simulink model "SEGWAY_SIM_PID"  (R2018a)
settings: Solver=ode23t  StartTime=0.0  StopTime=5  FixedStep=ts  RelTol=1e-6  AbsTol=1e-9
values from neighbouring files (symbols this model uses):
  param = [M m Ith Imr h W R Ke Rm Trmax Dm n]    [CONTROL_SEGWAY.m]
  X0 = [0 0 th0*pi/180]'    [CONTROL_SEGWAY.m]
undefined symbols (not defined in the file or in its folder): K, matA, matB, matC, matD, Td, Ti
settings Model: ExtModeTrigMode=oneshot  ExtModeArmWhenConnect=off  Creator=zamora  LastModifiedBy=zamora
settings SolverCC: AutoScaleAbsTol=off  ZeroCrossControl=EnableAll  ZeroCrossAlgorithm=Adaptive
settings DataIOCC: SaveFormat=Array  SignalLoggingSaveFormat=ModelDataLogs  SaveOutput=off  SaveTime=off  StateSaveName=x  TimeSaveName=t  OutputSaveName=y
settings OptimizationCC: BlockReduction=off  BooleanDataType=off  DefaultParameterBehavior=Inlined  BufferReuse=off  ExpressionDepthLimit=2147483647  LifeSpan=inf
settings DebuggingCC: SaveWithParameterizedLinksMsg=none  UnderspecifiedInitializationDetection=Classic  MergeDetectMultiDrivingBlocksExec=none  SignalResolutionControl=TryResolveAllWithWarning  MaxConsecutiveZCsMsg=none  IgnoredZcDiagnostic=none  MultiTaskDSMMsg=warning  MultiTaskCondExecSysMsg=none  FcnCallInpInsideContextMsg=warning  StateNameClashWarn=warning  SFUnexpectedBacktrackingDiag=warning  SFNoUnconditionalDefaultTransitionDiag=warning  SFExecutionAtInitializationDiag=none
settings HardwareCC: ProdBitPerPointer=32  ProdBitPerSizeT=32  ProdBitPerPtrDiffT=32  ProdLargestAtomicFloat=None  ProdIntDivRoundTo=Undefined  ProdEndianess=Unspecified  ProdWordSize=32  ProdHWDeviceType=32-bit Generic  TargetBitPerPointer=64  TargetBitPerSizeT=64  TargetBitPerPtrDiffT=64  TargetLongLongMode=on  TargetIntDivRoundTo=Zero  TargetEndianess=LittleEndian  TargetWordSize=64  TargetHWDeviceType=MATLAB Host  ProdEqTarget=off
settings ModelReferenceCC: PropagateSignalLabelsOutOfModel=off
settings RTWCC: TemplateMakefile=grt_unix.tmf
settings CodeAppCC: StateflowObjectComments=on
settings GRTTargetCC: TargetLangStandard=C89/C90 (ANSI)  GeneratePreprocessorConditionals=Disable all  CombineOutputUpdateFcns=off  GRTInterface=on
settings ConfigComp: CovMetricSettings=dw  CovHtmlReporting=on  CovSaveCumulativeToWorkspaceVar=on  CovSaveSingleToWorkspaceVar=on  CovExternalEMLEnable=off  CovSFcnEnable=off

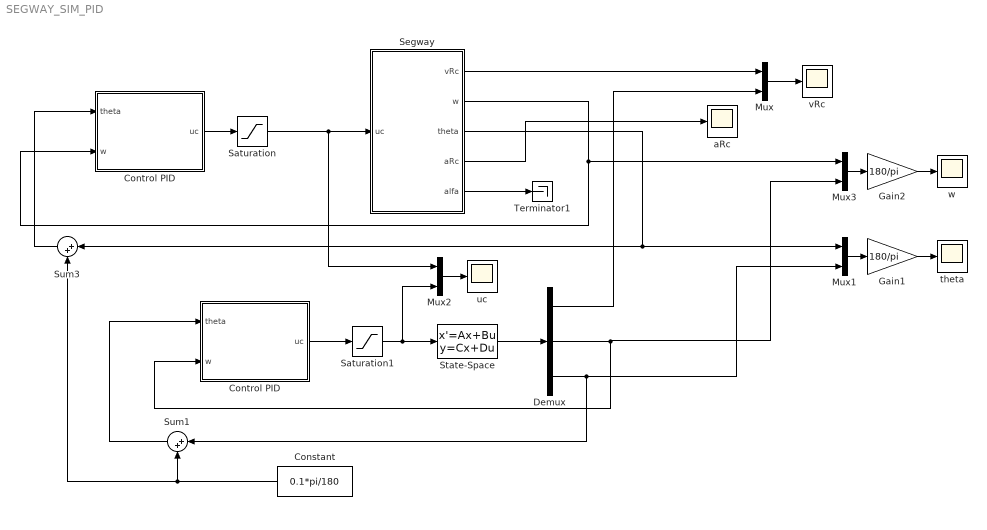
== system SEGWAY_SIM_PID ==
  Constant : Constant  Value=0.1*pi/180  SampleTime=0
  Control PID : Subsystem
  "Control PID " : Subsystem
  Demux : Demux  Outputs=3
  Gain1 : Gain  Gain=180/pi
  Gain2 : Gain  Gain=180/pi
  Mux{,1..3} (4 alike) : Mux  Inputs=2
  Saturation : Saturate  UpperLimit=8.5  LowerLimit=-8.5
  Saturation1 : Saturate  UpperLimit=8.5  LowerLimit=-8.5
  Segway : Subsystem
  State-Space : StateSpace  A=matA  B=matB  C=matC  D=matD  InitialCondition=X0
  Sum1 : Sum  Inputs=|++
  Sum3 : Sum  Inputs=|++
  Terminator1 : Terminator
  aRc : Scope
  theta : Scope
  uc : Scope
  vRc : Scope
  w : Scope
  wires:
  Gain1/1 -> theta/1
  Sum3/1 -> Control PID/1(theta)
  Control PID/1(uc) -> Saturation/1
  Segway/2(w) -> Control PID/2(w), Mux3/1
  Segway/5(alfa) -> Terminator1/1
  "Control PID "/1(uc) -> Saturation1/1
  Sum1/1 -> "Control PID "/1(theta)
  State-Space/1 -> Demux/1
  Demux/3 -> Mux1/2, Sum1/1
  Demux/2 -> Mux3/2, "Control PID "/2(w)
  Mux/1 -> vRc/1
  Mux1/1 -> Gain1/1
  Segway/4(aRc) -> aRc/1
  Saturation1/1 -> State-Space/1, Mux2/2
  Mux2/1 -> uc/1
  Segway/1(vRc) -> Mux/1
  Demux/1 -> Mux/2
  Segway/3(theta) -> Sum3/1, Mux1/1
  Saturation/1 -> Segway/1(uc), Mux2/1
  Constant/1 -> Sum3/2, Sum1/2
  Mux3/1 -> Gain2/1
  Gain2/1 -> w/1

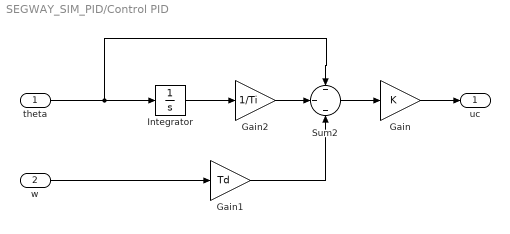
== system SEGWAY_SIM_PID/Control PID ==
  theta : Inport
  w : Inport  Port=2
  Gain : Gain  Gain=K
  Gain1 : Gain  Gain=Td
  Gain2 : Gain  Gain=1/Ti
  Integrator : Integrator
  Sum2 : Sum  Inputs=-|-|-
  uc : Outport
  wires:
  Gain/1 -> uc/1
  Gain1/1 -> Sum2/3
  Sum2/1 -> Gain/1
  Integrator/1 -> Gain2/1
  Gain2/1 -> Sum2/2
  theta/1 -> Integrator/1, Sum2/1
  w/1 -> Gain1/1

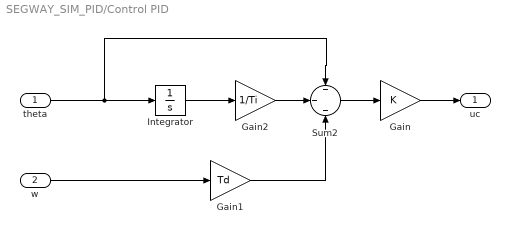
== system SEGWAY_SIM_PID/Control PID  ==
  theta : Inport
  w : Inport  Port=2
  Gain : Gain  Gain=K
  Gain1 : Gain  Gain=Td
  Gain2 : Gain  Gain=1/Ti
  Integrator : Integrator
  Sum2 : Sum  Inputs=-|-|-
  uc : Outport
  wires:
  Gain/1 -> uc/1
  Gain1/1 -> Sum2/3
  Sum2/1 -> Gain/1
  Integrator/1 -> Gain2/1
  Gain2/1 -> Sum2/2
  theta/1 -> Integrator/1, Sum2/1
  w/1 -> Gain1/1

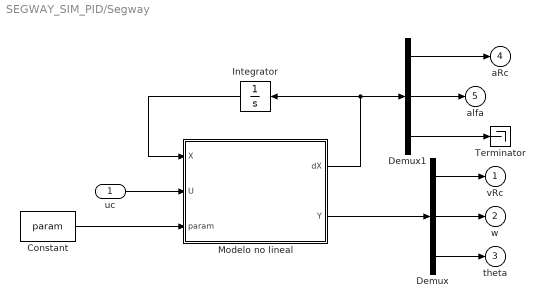
== system SEGWAY_SIM_PID/Segway ==
  uc : Inport  SampleTime=0
  Constant : Constant  Value=param  SampleTime=0
  Demux : Demux  Outputs=3
  Demux1 : Demux  Outputs=3
  Integrator : Integrator  InitialCondition=X0
  Modelo no lineal : MATLAB Function  TreatAsAtomicUnit=on
  Terminator : Terminator
  vRc : Outport  InitialOutput=0
  w : Outport  Port=2  InitialOutput=0
  theta : Outport  Port=3  InitialOutput=0
  aRc : Outport  Port=4  InitialOutput=0
  alfa : Outport  Port=5  InitialOutput=0
  wires:
  Modelo no lineal/1(dX) -> Demux1/1, Integrator/1
  Integrator/1 -> Modelo no lineal/1(X)
  Constant/1 -> Modelo no lineal/3(param)
  uc/1 -> Modelo no lineal/2(U)
  Demux/1 -> vRc/1
  Demux/2 -> w/1
  Demux/3 -> theta/1
  Modelo no lineal/2(Y) -> Demux/1
  Demux1/2 -> alfa/1
  Demux1/3 -> Terminator/1
  Demux1/1 -> aRc/1

== matlab function SEGWAY_SIM_PID/Segway/Modelo no lineal ==
  data: X input; dX output; U input; param input; Y output
function [dX,Y] = segway(X,U,param)

%% Parametros
% Masa del chasis (kg)
M=param(1);
% Masa de la rueda incluyendo el rotor del motor (kg)
m=param(2);
% Momento de inercia de cabeceo del chasis (kg.m^2)
Ith=param(3);
% Momento de inercia del conjunto motor + rueda (kg.m^2)
Imr=param(4);
% Distancia al centro de gravedad del chasis medida desde el eje (m)
h=param(5);
% Distancia de separacion entre ruedas (m)
W=param(6);
% Radio de las rueda (m)
R=param(7);
% Constante electrica del motor (V.s/rad)
Ke=param(8);
% Constante mecanica del motor (N.m/A)
Kt=Ke;
% Resistencia electrica del motor
Rm=param(9);
% Par de friccion del motor (N.m) eje externo
Trmax=param(10);
% Coeficiente de friccion viscosa eje externo (N.m.s/rad)
Dm=param(11);
% Relacion de engranajes
n=param(12);


% Gravedad (m/s^2)
g=9.81;

%% Entradas
% Tension comun (V)
uc=U(1);

%% Variables de estado
% Velocidad comun lineal de las ruedas (m/s)
vRc=X(1);
% Velocidad angular de cabeceo (rad/s)
wth=X(2);
% Angulo de cabeceo (rad)
th=X(3);
% Velocidad angular de la rueda (rad/s)
wRc=vRc/R;
% Velocidad angular del motor
wmc=n*wRc-wth;


%% Motor
% Ecuacion electrica del motor
ic=(uc-Ke*wmc)/Rm;
% Par motor eje motor
Tmc=Kt*ic;
% Par motor límite (eje motor) para aplicación del par máximo de fricción (eje rueda)
wmc_aux = 5*[-2 -1 1 2];
Trc_aux = Trmax/n*[-1 -1 1 1];
% Tmc_lim=Tmc*(Tmc>-Trmax/n && Tmc<Trmax/n)-Trmax/n*(Tmc<=-Trmax/n)+Trmax*(Tmc>=Trmax/n);
% Par de friccion estatico (eje rueda)
% Trc=n*Tmc_lim*(abs(wmc)==0)+Trmax*sign(wmc)*(abs(wmc)>0);
Trc = interp1(wmc_aux,Trc_aux,wmc,'linear','extrap');
% Par neto (eje motor)
Tc=Tmc-Dm*wRc/n-Trc/n;

%% Avance del vehiculo y cabeceo
% 2*n*Tc/R = (2*(m+Imr/R^2)+M)*aRc + M*h*alfath*cos(th) - M*wth^2*h*sin(th)
% -2*Tc + M*g*h*sin(th) = M*h*cos(th)*aRc + (Ith+M*h^2)*alfath
% Se resuelve el sistema de ecuaciones anterior
matA_aux=[2*(m+Imr/R^2)+M   M*h*cos(th)
              M*h*cos(th)   Ith+M*h^2];
matB_aux=[2*n*Tc/R + M*wth^2*h*sin(th) ; -2*Tc + M*g*h*sin(th)];
aux=matA_aux\matB_aux;
aRc=aux(1);
alfath=aux(2); 

% Derivada del vector de estado
dX=[aRc alfath wth]';

%% Ecuaciones de salida
Y = X;
